simulink model "stm32f4_ds3231_read_temperature_demo"  (Simulink 7.3)
settings: Solver=FixedStepDiscrete  SolverMode=SingleTasking  StartTime=0.0  StopTime=10.0  RelTol=1e-3
PreLoadFcn:
  | waijung.modelPreload; % Required for working with Waijung Blockset. Do not remove.
undefined symbols (not defined in the file): HSEOSC, Link, LQFP176, ST, STM32F417IG
libraries: simulink x5, stm32f4_device_config_lib x1
CloseFcn:
  | waijung.modelClose; % Required for working with Waijung Blockset. Do not remove.
settings Model: Creator=Krisada  LastModifiedBy=Krisada
settings OptimizationCC: OptimizeModelRefInitCode=on  LifeSpan=1
settings HardwareCC: ProdEndianess=LittleEndian  ProdHWDeviceType=ARM Compatible->Cortex - M4  TargetEndianess=LittleEndian  TargetHWDeviceType=ARM Compatible->Cortex - M4
settings RTWCC: SystemTargetFile=stm32f4.tlc  GenerateMakefile=off  TemplateMakefile=ert_default_tmf  Description=STM32F4 Target  ProcessScript=stm32f4_make_rtw_hook
settings CodeAppCC: IgnoreCustomStorageClasses=off
settings STFCustomTargetCC: ModelReferenceCompliant=off  CombineOutputUpdateFcns=on  ERTCustomFileBanners=on  SupportContinuousTime=off  SupportNonInlinedSFcns=off  SystemTargetFile=stm32f4.tlc
settings ERTTargetCC: MultiwordLength=2048  ModelReferenceCompliant=off  ParMdlRefBuildCompliant=off  CompOptLevelCompliant=off  ERTFirstTimeCompliant=off  ModelStepFunctionPrototypeControlCompliant=off  CPPClassGenCompliant=off  ExtModeMexFile=noextcomm  InlinedParameterPlacement=NonHierarchical  ERTSrcFileBannerTemplate=stm32f4_code_template.cgt  ERTHdrFileBannerTemplate=stm32f4_code_template.cgt  ERTDataSrcFileTemplate=stm32f4_code_template.cgt  ERTDataHdrFileTemplate=stm32f4_code_template.cgt  ERTCustomFileTemplate=stm32f4_file_process.tlc

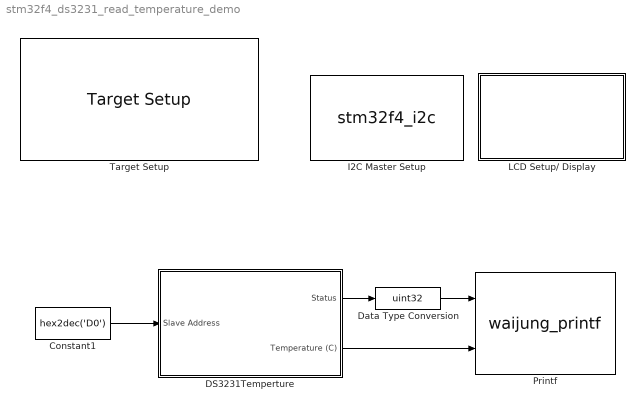
== system stm32f4_ds3231_read_temperature_demo ==
  Constant1 : Constant  Value=hex2dec('D0')  OutDataTypeMode=uint8  OutDataType=fixdt(1, 16)  OutScaling=2^0  OutDataTypeStr=uint8  SampleTime=0.5
  DS3231Temperture : Subsystem  mask{blockfunction=temp, module=1}
      mask prompts: blockfunction "Function"; module "I2C module"
      mask help:
      | The block implement temperature reading from DS3231 (Extremely Accurate RTC).
      | Its override the CONV bit, to force the temperature update, so the recommend sample time for this block is more than 0.5 seconds.
      | To get reading value from DS3231 device, this block generate 3 transaction of I2C as below:
      | 1. Read 2 bytes data from register 0x11 and 0x12 (Sequential read).
      | 2. Read 1 byte data from register 0x0F (Status) for poll BSY bit.
      | 3. Write 1 byte data to register 0x0E to force temperature conversion, CONV bit.
      mask init:
      | amg_high_precision_rtc_callback('init');
      mask StyleString: popup(temp|time|date),popup(1|2|3)
      mask CallbackString: |amg_high_precision_rtc_callback('module');
      mask Display: text(0.5, 0.5, 'Port: I2C1','ver','middle','hor','center');port_label('input', 1,'SlvAddr');port_label('output', 1,'Status');port_label('output', 2,'Temp (C)');
  Data Type Conversion : DataTypeConversion  OutDataTypeMode=uint32  OutDataType=fixdt(1, 16)  OutScaling=2^0  OutDataTypeStr=uint32
  I2C Master Setup : S-Function  FunctionName=stm32f4_i2c  Parameters=configuration,module,transfer,clkspeed,timeout,sdapin,sclpin,writecount,readcount,inputtypearray,outputtypearray,confstr,sampletime,sampletimestr,blockid  EnableBusSupport=off  mask(stm32f4_i2c){configuration=Setup, module=1, lastmodule=1, transfer=Blocking, dutycycle=TLow/THigh = 2, clkspeed=400, timeout=25, writecount=0, readcount=0, sdapin=B7, sclpin=B6, waitwritetime=0, inputtypearray=[0], outputtypearray=[0], confstr=["B","7","B","6","1","1","6","0","I2C_DutyCycle_2","0","off"], sampletime=-1, sampletimestr=0.01, blockid=I2CMasterSetup}
      mask prompts: module "I2C Module"; lastmodule "Last module"; transfer "Transfer mode"; dutycycle "Duty cycle in fast mode"; clkspeed "Clock speed (kHz)"; timeout "Timeout (ms)"; writecount "Bytes write count"; readcount "Bytes read count"; sdapin "SDA pin"; sclpin "SCL pin"; waitwritetime "Wait write time (ms), default is 0"; inputtypearray "Input type array"; outputtypearray "Output type array"; confstr "Configuration string"; sampletime "Sample time (sec)"; sampletimestr "Compiled sample time (sec) in string"
      mask init:
      | stm32f4_i2c_callback('init');
      mask Help: web(fullfile(waijungdocroot,'stm32f4_i2c_setup.htm'), '-browser')
      mask StyleString: popup(Setup|Transaction),popup(1|2|3),edit,popup(Blocking|Non-blocking),popup(TLow/THigh = 16/9|TLow/THigh = 2),edit,edit,edit,edit,popup(Not used|B7|B9),popup(Not used|B6|B8),edit,edit,edit,edit,edit,edit,edit
      mask CallbackString: stm32f4_i2c_callback('configuration');|stm32f4_i2c_callback('module');|||stm32f4_i2c_callback('dutycycle');|||stm32f4_i2c_callback('writecount');|stm32f4_i2c_callback('readcount');|stm32f4_i2c_callback('sdapin');|stm32f4_i2c_callback('sclpin');||||stm32f4_i2c_callback('confstr');|stm32f4_i2c_callback('sampletime');|stm32f4_i2c_callback('sampletimestr');|stm32f4_i2c_callback('blockid');
      mask Display: text(0.5, 0.5, 'Module: I2C1\nClock: 400kHz\nSDA/SCL Pin: B7/B6','ver','middle','hor','center');
  LCD Setup/ Display : Subsystem
  Printf : S-Function  FunctionName=waijung_printf  Parameters=storagename,printfformat,formatcode,varname,sampletime,sampletimestr,blockid  EnableBusSupport=off  mask(waijung_printf){storagename=S, printfformat=Status:%u, %1.2fC, formatcode=uf, varname=LCDSetupDisplayVolatileDataStorage_S, sampletime=-1, sampletimestr=0.5, blockid=Printf}
      mask prompts: storagename "Storage Name"; printfformat "Printf format"; formatcode "Printf format code"; varname "Variable name"; sampletime "Sample time (sec)"; sampletimestr "Compiled sample time (sec) in string"
      mask help: This block implements printf command.
      mask init:
      | waijung_printf_callback('init');
      mask Help: web(fullfile(waijungdocroot,'waijung_printf.htm'))
      mask StyleString: popup(S),edit,edit,edit,edit,edit,edit
      mask CallbackString: waijung_printf_callback('storagename');|waijung_printf_callback('printfformat');|waijung_printf_callback('formatcode');|waijung_printf_callback('varname');|waijung_printf_callback('sampletime');|waijung_printf_callback('sampletimestr');|waijung_printf_callback('blockid');
      mask Display: text(0.95, 0.5, 'Buffer: S\nTs (sec): 0.5','ver','middle','hor','right');port_label('input',1,'D1(%u)');port_label('input',2,'D2(%f)');
  Target Setup : stm32f4_device_config_lib/Target Setup  Priority=100  compiler=GNU ARM  previous_compiler=GNU ARM  mcu=STM32F417IG (LQFP176)  mcustr=STM32F417IG  clockconfig=HSEOSC-8MHz  system_stm32f4xx_c_path=F:\trunk\targets\stm32f4_target\stm32f4\utils\system_stm32f4xx_default\STM32F40_41xxx\hseosc8mhz  showmemoryconfiguration=off  stacksize=0x400  heapsize=0x200  enableautocompiledownload=on  fullchiperase=off  programmerinterface=ST-Link  editctrlstr=on  compilercontrolstr=$(patsubst %, -I%, .) -mcpu=cortex-m4 -mthumb -mthumb-interwork -mfloat-abi=hard -mfpu=fpv4-sp-d16 -ffast-math -Wall -Wextra -Ofast  assemblercontrolstr=$(patsubst %, -I%, .) -mcpu=cortex-m4 -mthumb -mthumb-interwork -mfloat-abi=hard -mfpu=fpv4-sp-d16 -ffast-math -Wall -Wextra -Ofast -Wa,-amhls=$(<:.s=.lst) -D__STACK_SIZE=$(STACK_SIZE) -D__HEAP_SIZE=$(HEAP_SIZE)  linkercontrolstr=-T$(LD_SCRIPT) -g -Wl,-Map=$(MAP),--cref,--no-warn-mismatch -mcpu=cortex-m4 -mthumb -mthumb-interwork -mfloat-abi=hard -mfpu=fpv4-sp-d16 -specs=nosys.specs  runafterdownload=on  execprofile=None  profileruart=1  profilerbaud=115200  profilertxpin=D8  profilerinitstr=0.01,168000000,1680000,115200,0  manualsetsampletime=off  sampletime=0.01  blockid=TargetSetup  systickreloadvalue=1680000  hseval=8000000  lastprofileruart=1  hclk=168000000  flashorigin=0x8000000  flashlength=1024k  ramorigin=0x20000000  ramlength=128k  useextram=off
  wires:
  Data Type Conversion/1 -> Printf/1
  DS3231Temperture/2(Temperature (C)) -> Printf/2
  DS3231Temperture/1(Status) -> Data Type Conversion/1
  Constant1/1 -> DS3231Temperture/1(Slave Address)

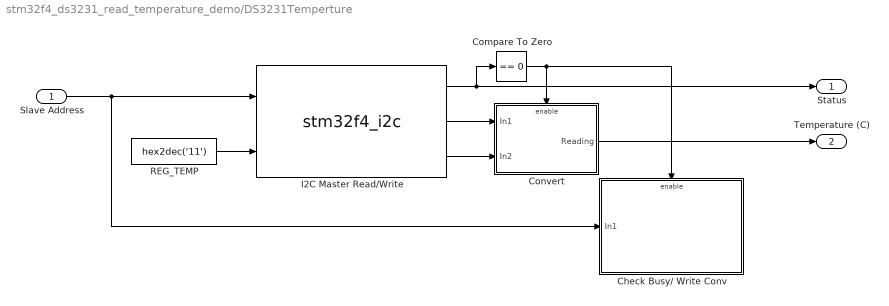
== system stm32f4_ds3231_read_temperature_demo/DS3231Temperture ==
  Slave Address : Inport  OutDataType=fixdt(1, 16)  OutScaling=2^0
  Check Busy/ Write Conv : Subsystem
  Compare To Zero : simulink/Logic and Bit Operations/Compare To Zero  SystemSampleTime=-1  relop===  LogicOutDataTypeMode=uint8  ZeroCross=off
  Convert : Subsystem  TreatAsAtomicUnit=on
  I2C Master Read/Write : S-Function  FunctionName=stm32f4_i2c  Parameters=configuration,module,transfer,clkspeed,timeout,sdapin,sclpin,writecount,readcount,inputtypearray,outputtypearray,confstr,sampletime,sampletimestr,blockid  EnableBusSupport=off  mask(stm32f4_i2c){configuration=Transaction, module=1, lastmodule=3, transfer=Blocking, dutycycle=TLow/THigh = 2, clkspeed=400, timeout=25, writecount=1, readcount=2, sdapin=C9, sclpin=A8, waitwritetime=0, inputtypearray=[2 3 3], outputtypearray=[3 3 3 3], confstr=["C","9","A","8","1","1","6","0","I2C_DutyCycle_2","0","off"], sampletime=-1, sampletimestr=0.5, blockid=DS3231TempertureI2CMasterReadWrite}
      mask prompts: module "I2C Module"; lastmodule "Last module"; transfer "Transfer mode"; dutycycle "Duty cycle in fast mode"; clkspeed "Clock speed (kHz)"; timeout "Timeout (ms)"; writecount "Bytes write count"; readcount "Bytes read count"; sdapin "SDA pin"; sclpin "SCL pin"; waitwritetime "Wait write time (ms), default is 0"; inputtypearray "Input type array"; outputtypearray "Output type array"; confstr "Configuration string"; sampletime "Sample time (sec)"; sampletimestr "Compiled sample time (sec) in string"
      mask init:
      | stm32f4_i2c_callback('init');
      mask Help: web(fullfile(waijungdocroot,'stm32f4_i2c_readwrite.htm'), '-browser')
      mask StyleString: popup(Setup|Transaction),popup(1|2|3),edit,popup(Blocking|Non-blocking),popup(TLow/THigh = 16/9|TLow/THigh = 2),edit,edit,edit,edit,popup(-|C9),popup(-|A8),edit,edit,edit,edit,edit,edit,edit
      mask CallbackString: stm32f4_i2c_callback('configuration');|stm32f4_i2c_callback('module');|||stm32f4_i2c_callback('dutycycle');|||stm32f4_i2c_callback('writecount');|stm32f4_i2c_callback('readcount');|stm32f4_i2c_callback('sdapin');|stm32f4_i2c_callback('sclpin');||||stm32f4_i2c_callback('confstr');|stm32f4_i2c_callback('sampletime');|stm32f4_i2c_callback('sampletimestr');|stm32f4_i2c_callback('blockid');
      mask Display: text(0.5, 0.5, 'Module: I2C1\nTransfer: Blocking\nWrite: 1 bytes\nRead: 2 bytes\nTs (sec): 0.5','ver','middle','hor','center');port_label('input', 1,'SlvAddr');port_label('input', 2,'Wr0 (uint8)');port_label('output', 1,'Status');port_label('output', 2,'Rd0 (uint8)');port_label('output', 3,'Rd1 (uint8)');
  REG_TEMP : Constant  Value=hex2dec('11')  OutDataTypeMode=uint8  OutDataType=fixdt(1, 16)  OutScaling=2^0  OutDataTypeStr=uint8
  Status : Outport
  Temperature (C) : Outport  Port=2
  wires:
  Convert/1(Reading) -> Temperature (C)/1
  I2C Master Read/Write/3 -> Convert/2(In2)
  I2C Master Read/Write/2 -> Convert/1(In1)
  Compare To Zero/1 -> Check Busy/ Write Conv/Enable, Convert/Enable
  I2C Master Read/Write/1 -> Compare To Zero/1, Status/1
  REG_TEMP/1 -> I2C Master Read/Write/2
  Slave Address/1 -> Check Busy/ Write Conv/1(In1), I2C Master Read/Write/1

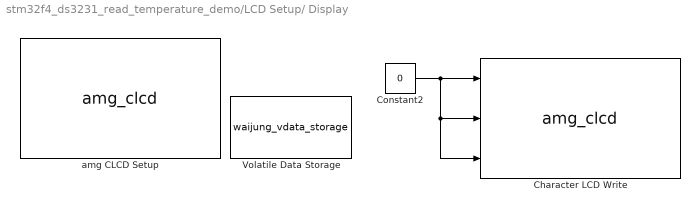
== system stm32f4_ds3231_read_temperature_demo/LCD Setup/ Display ==
  Character LCD Write : S-Function  FunctionName=amg_clcd  Parameters=module,configuration,inputtypearray,outputtypearray,confstr,sampletime,sampletimestr,blockid  EnableBusSupport=off  mask(amg_clcd){configuration=Transaction, module=1, model=amg CLCD Std, interface=4-bits, linecount=4, columncount=20, gpiotype=Push-pull, controlport=E, control_rs=15, control_rw=13, control_en=11, dataport=A, data0=7, data1=5, data2=3, data3=1, usestringbuffer=on, stringbuffer=S, varname=LCDSetupDisplayVolatileDataStorage_S, inputtypearray=[3 -1 -1 -1], outputtypearray=[0], confstr=["4","4","20","PP","E","15","11","13","","A","","","","","7","5","3","1","1","LCDSetupDisplayVolatileDataStorage_S","1","0","0","0","1","0","0","0","0","stm32f4"], sampletime=-1, sampletimestr=0.01, blockid=LCDSetupDisplayCharacterLCDWrite}
      mask prompts: model "LCD model:"; linecount "Number of lines:"; columncount "Number of columns:"; gpiotype "GPIO Output type:"; controlport "GPIO control port:"; control_rs "GPIO control pin, RS:"; control_rw "GPIO control pin, RW:"; control_en "GPIO control pin, EN:"; dataport "GPIO data D[7:4] port"; data0 "GPIO data pin, D4:"; data1 "GPIO data pin, D5:"; data2 "GPIO data pin, D6:"; data3 "GPIO data pin, D7:"; usestringbuffer "Use string buffer"; stringbuffer "String buffer"; varname "Variable name"; inputtypearray "Input type array"; outputtypearray "Output type array"; confstr "Configuration string"; sampletime "Sample time (sec)"; sampletimestr "Compiled sample time (sec) in string"
      mask help:
      | Note for cmd:
      | 1 - Clear LCD Line before write.
      | 0 or otherwise - Write into LCD Line with existing data.
      mask init:
      | amg_clcd_callback('init');
      mask Help: web(fullfile(waijungdocroot,'amg_clcd_write.htm'), '-browser')
      mask StyleString: popup(Setup|Transaction),popup(1|2|3|4),popup(amg CLCD Std),popup(4-bits),edit,edit,popup(Push-pull|Open-drain),popup(A|B|C|D|E|F|G|H|I),popup(0|1|2|3|4|5|6|7|8|9|10|11|12|13|14|15),popup(0|1|2|3|4|5|6|7|8|9|10|11|12|13|14|15),popup(0|1|2|3|4|5|6|7|8|9|10|11|12|13|14|15),popup(A|B|C|D|E|F|G|H|I),popup(0|1|2|3|4|5|6|7|8|9|10|11|12|13|14|15),popup(0|1|2|3|4|5|6|7|8|9|10|11|12|13|14|15),popup(0|1|2|3|4|5|6|7|8|9|10|11|12|13|14|15),popup(0|1|2|3|4|5|6|7|8|9|10|11|12|13|14|15),checkbox,popup(S),edit,edit,edit,edit,edit,edit,edit
      mask CallbackString: amg_clcd_callback('configuration');||||||||||||||||amg_clcd_callback('usestringbuffer');||amg_clcd_callback('varname');|||amg_clcd_callback('confstr');|amg_clcd_callback('sampletime');|amg_clcd_callback('sampletimestr');|amg_clcd_callback('blockid');
      mask Display: text(0.5, 0.5, 'Module: CLCD1 (Write)\nBuffer: S\nTs (sec): 0.01','ver','middle','hor','center');port_label('input', 1,'cmd');port_label('input', 2,'xpos');port_label('input', 3,'ypos');
  Constant2 : Constant  Value=0  OutDataTypeMode=uint8  OutDataType=fixdt(1, 16)  OutScaling=2^0  OutDataTypeStr=uint8
  Volatile Data Storage : S-Function  FunctionName=waijung_vdata_storage  Parameters=storagetype,storagename,initval,varname,buffersize,initvalstring,sampletime,sampletimestr,blockid,storagetypestr  EnableBusSupport=off  mask(waijung_vdata_storage){storagetype=string, storagename=S, initval=0, varname=LCDSetupDisplayVolatileDataStorage_S, buffersize=64, initvalstring='', webintegration=Disable, weboutputformat='%s', webcgicallback=(void*)0, laststoragetype=string, sampletime=-1, sampletimestr=0.01, blockid=LCDSetupDisplayVolatileDataStorage, storagetypestr=char}
      mask prompts: storagetype "Storage Type"; storagename "Storage Name (must be a valid variable name)"; initval "Initial value (Apply at Power on Reset only)"; varname "Variable name"; buffersize "Size (bytes)"; initvalstring "Initial value (Apply at Power on Reset only)"; webintegration "Web CGI varget/varset integration"; weboutputformat "Web CGI varget output format"; webcgicallback "Web CGI varset callback"; laststoragetype "Last selected Storage Type"; sampletime "Sample time (sec)"; sampletimestr "Compiled sample time (sec) in string"; storagetypestr "Type string"
      mask help:
      | This block implements a volatile Data Storage.
      |
      | Web CGI varset/varget integratiopn:
      | Enable - In webserver application, allow remote access via http.
      | Disable - Variable is use in local only.
      mask init:
      | waijung_vdata_storage_callback('init');
      mask Help: web(fullfile(waijungdocroot,'Volatile_Data_Storage.htm'))
      mask StyleString: popup(double|single|uint32|int32|uint16|int16|uint8|int8|string),edit,edit,edit,edit,edit,popup(Disable|ReadOnly|Write/ Read|ReadOnly with KeyValuePair|Write/ Read with KeyValuePair),edit,edit,popup(double|single|uint32|int32|uint16|int16|uint8|int8|string),edit,edit,edit,edit
      mask CallbackString: waijung_vdata_storage_callback('storagetype');|waijung_vdata_storage_callback('storagename');|waijung_vdata_storage_callback('initval');|waijung_vdata_storage_callback('varname');||waijung_vdata_storage_callback('initvalstring');|waijung_vdata_storage_callback('webintegration');|waijung_vdata_storage_callback('weboutputformat');|||waijung_vdata_storage_callback('sampletime');|waijung_vdata_storage_callback('sampletimestr');|waijung_vdata_storage_callback('blockid');|
      mask Display: text(0.5, 0.5, 'Name: S\nType: string','ver','middle','hor','center')
  amg CLCD Setup : S-Function  FunctionName=amg_clcd  Parameters=module,configuration,inputtypearray,outputtypearray,confstr,sampletime,sampletimestr,blockid  EnableBusSupport=off  mask(amg_clcd){configuration=Setup, module=1, model=amg CLCD Std, interface=4-bits, linecount=4, columncount=16, gpiotype=Push-pull, controlport=E, control_rs=7, control_rw=8, control_en=9, dataport=E, data0=12, data1=13, data2=14, data3=15, usestringbuffer=off, stringbuffer=Line2, varname=clcd_demo_4linesLCDSetupVolatileDataStorage3_Line2, inputtypearray=[0], outputtypearray=[0], confstr=["4","4","16","PP","E","7","9","8","","E","","","","","12","13","14","15","0","","0","0","0","0","1","0","0","0","0","stm32f4"], sampletime=-1, sampletimestr=0.01, blockid=LCDSetupDisplayamgCLCDSetup}
      mask prompts: model "LCD model:"; linecount "Number of lines:"; columncount "Number of columns:"; gpiotype "GPIO Pull-Up/Down:"; controlport "GPIO control port:"; control_rs "GPIO control pin, RS:"; control_rw "GPIO control pin, RW:"; control_en "GPIO control pin, EN:"; dataport "GPIO data D[7:4] port"; data0 "GPIO data pin, D4:"; data1 "GPIO data pin, D5:"; data2 "GPIO data pin, D6:"; data3 "GPIO data pin, D7:"; usestringbuffer "Use string buffer"; stringbuffer "String buffer"; varname "Variable name"; inputtypearray "Input type array"; outputtypearray "Output type array"; confstr "Configuration string"; sampletime "Sample time (sec)"; sampletimestr "Compiled sample time (sec) in string"
      mask init:
      | amg_clcd_callback('init');
      mask Help: web(fullfile(waijungdocroot,'amg_clcd_setup.htm'), '-browser')
      mask StyleString: popup(Setup|Transaction),popup(1|2|3|4),popup(amg CLCD Std),popup(4-bits),edit,edit,popup(Push-pull|Open-drain),popup(A|B|C|D|E|F|G|H|I),popup(0|1|2|3|4|5|6|7|8|9|10|11|12|13|14|15),popup(0|1|2|3|4|5|6|7|8|9|10|11|12|13|14|15),popup(0|1|2|3|4|5|6|7|8|9|10|11|12|13|14|15),popup(A|B|C|D|E|F|G|H|I),popup(0|1|2|3|4|5|6|7|8|9|10|11|12|13|14|15),popup(0|1|2|3|4|5|6|7|8|9|10|11|12|13|14|15),popup(0|1|2|3|4|5|6|7|8|9|10|11|12|13|14|15),popup(0|1|2|3|4|5|6|7|8|9|10|11|12|13|14|15),checkbox,popup(Line3|Line1|Line2|Line4),edit,edit,edit,edit,edit,edit,edit
      mask CallbackString: amg_clcd_callback('configuration');||||||||||||||||amg_clcd_callback('usestringbuffer');||amg_clcd_callback('varname');|||amg_clcd_callback('confstr');|amg_clcd_callback('sampletime');|amg_clcd_callback('sampletimestr');|amg_clcd_callback('blockid');
      mask Display: text(0.5, 0.5, 'Module: CLCD1 (Setup)\nInterface: 4-bits\nCntrl: E7/E8/E9\nD[7:4]: E12/E13/E14/E15\nTs (sec): 0.01','ver','middle','hor','center');
  wires:
  Constant2/1 -> Character LCD Write/1, Character LCD Write/2, Character LCD Write/3

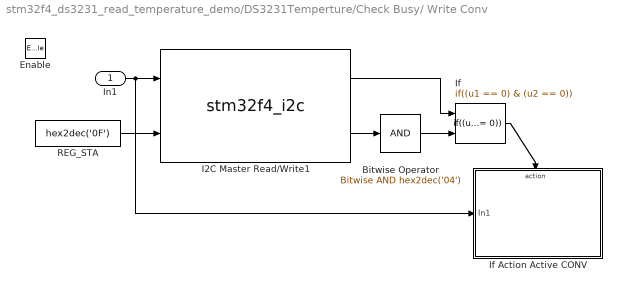
== system stm32f4_ds3231_read_temperature_demo/DS3231Temperture/Check Busy/ Write Conv ==
  In1 : Inport
  Enable : EnablePort
  Bitwise Operator : simulink/Logic and Bit Operations/Bitwise Operator  logicop=AND  UseBitMask=on  BitMask=hex2dec('04')  BitMaskRealWorld=Stored Integer
  I2C Master Read/Write1 : S-Function  FunctionName=stm32f4_i2c  Parameters=configuration,module,transfer,clkspeed,timeout,sdapin,sclpin,writecount,readcount,inputtypearray,outputtypearray,confstr,sampletime,sampletimestr,blockid  EnableBusSupport=off  mask(stm32f4_i2c){configuration=Transaction, module=1, lastmodule=3, transfer=Blocking, dutycycle=TLow/THigh = 2, clkspeed=400, timeout=25, writecount=1, readcount=1, sdapin=C9, sclpin=A8, waitwritetime=0, inputtypearray=[2 3 3], outputtypearray=[2 3 3], confstr=["C","9","A","8","1","1","6","0","I2C_DutyCycle_2","0","off"], sampletime=-1, sampletimestr=0.5, blockid=DS3231TempertureCheckBusyWriteConvI2CMasterReadWrite1}
      mask prompts: module "I2C Module"; lastmodule "Last module"; transfer "Transfer mode"; dutycycle "Duty cycle in fast mode"; clkspeed "Clock speed (kHz)"; timeout "Timeout (ms)"; writecount "Bytes write count"; readcount "Bytes read count"; sdapin "SDA pin"; sclpin "SCL pin"; waitwritetime "Wait write time (ms), default is 0"; inputtypearray "Input type array"; outputtypearray "Output type array"; confstr "Configuration string"; sampletime "Sample time (sec)"; sampletimestr "Compiled sample time (sec) in string"
      mask init:
      | stm32f4_i2c_callback('init');
      mask Help: web(fullfile(waijungdocroot,'stm32f4_i2c_readwrite.htm'), '-browser')
      mask StyleString: popup(Setup|Transaction),popup(1|2|3),edit,popup(Blocking|Non-blocking),popup(TLow/THigh = 16/9|TLow/THigh = 2),edit,edit,edit,edit,popup(-|C9),popup(-|A8),edit,edit,edit,edit,edit,edit,edit
      mask CallbackString: stm32f4_i2c_callback('configuration');|stm32f4_i2c_callback('module');|||stm32f4_i2c_callback('dutycycle');|||stm32f4_i2c_callback('writecount');|stm32f4_i2c_callback('readcount');|stm32f4_i2c_callback('sdapin');|stm32f4_i2c_callback('sclpin');||||stm32f4_i2c_callback('confstr');|stm32f4_i2c_callback('sampletime');|stm32f4_i2c_callback('sampletimestr');|stm32f4_i2c_callback('blockid');
      mask Display: text(0.5, 0.5, 'Module: I2C1\nTransfer: Blocking\nWrite: 1 bytes\nRead: 1 bytes\nTs (sec): 0.5','ver','middle','hor','center');port_label('input', 1,'SlvAddr');port_label('input', 2,'Wr0 (uint8)');port_label('output', 1,'Status');port_label('output', 2,'Rd0 (uint8)');
  If : If  NumInputs=2  IfExpression=(u1 == 0) & (u2 == 0)  ShowElse=off
  If Action Active CONV : Subsystem  TreatAsAtomicUnit=on
  REG_STA : Constant  Value=hex2dec('0F')  OutDataTypeMode=uint8  OutDataType=fixdt(1, 16)  OutScaling=2^0  OutDataTypeStr=uint8
  wires:
  If/1 -> If Action Active CONV/Action
  Bitwise Operator/1 -> If/2
  I2C Master Read/Write1/2 -> Bitwise Operator/1
  In1/1 -> If Action Active CONV/1(In1), I2C Master Read/Write1/1
  I2C Master Read/Write1/1 -> If/1
  REG_STA/1 -> I2C Master Read/Write1/2

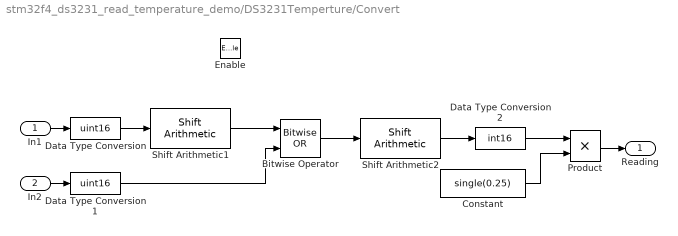
== system stm32f4_ds3231_read_temperature_demo/DS3231Temperture/Convert ==
  In1 : Inport  OutDataType=fixdt(1, 16)  OutScaling=2^0
  In2 : Inport  Port=2  OutDataType=fixdt(1, 16)  OutScaling=2^0
  Enable : EnablePort
  Bitwise Operator : simulink/Logic and Bit Operations/Bitwise Operator  logicop=OR  UseBitMask=off  NumInputPorts=2  BitMask=bin2dec('11011001')  BitMaskRealWorld=Stored Integer
  Constant : Constant  Value=single(0.25)  OutDataType=fixdt(1, 16)  OutScaling=2^0
  Data Type Conversion : DataTypeConversion  OutDataTypeMode=uint16  OutDataType=fixdt(1, 16)  OutScaling=2^0  OutDataTypeStr=uint16
  Data Type Conversion1 : DataTypeConversion  OutDataTypeMode=uint16  OutDataType=fixdt(1, 16)  OutScaling=2^0  OutDataTypeStr=uint16
  Data Type Conversion2 : DataTypeConversion  OutDataTypeMode=int16  OutDataType=fixdt(1, 16)  OutScaling=2^0  OutDataTypeStr=int16
  Product : Product  OutDataTypeMode=single  OutDataType=fixdt(1, 16)  OutScaling=2^0  OutDataTypeStr=single  RndMeth=Zero
  Shift Arithmetic1 : simulink/Logic and Bit Operations/Shift Arithmetic  SystemSampleTime=-1  nBitShiftRight=-8  nBinPtShiftRight=0
  Shift Arithmetic2 : simulink/Logic and Bit Operations/Shift Arithmetic  SystemSampleTime=-1  nBitShiftRight=6  nBinPtShiftRight=0
  Reading : Outport  OutDataType=fixdt(1, 16)  OutScaling=2^0
  wires:
  Shift Arithmetic2/1 -> Data Type Conversion2/1
  Product/1 -> Reading/1
  Constant/1 -> Product/2
  Data Type Conversion2/1 -> Product/1
  Bitwise Operator/1 -> Shift Arithmetic2/1
  Data Type Conversion1/1 -> Bitwise Operator/2
  Shift Arithmetic1/1 -> Bitwise Operator/1
  Data Type Conversion/1 -> Shift Arithmetic1/1
  In2/1 -> Data Type Conversion1/1
  In1/1 -> Data Type Conversion/1

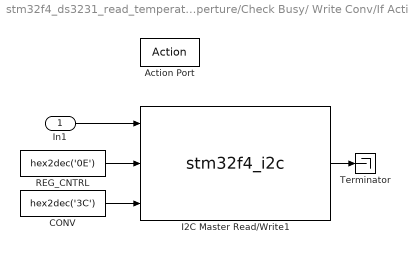
== system stm32f4_ds3231_read_temperature_demo/DS3231Temperture/Check Busy/ Write Conv/If Action Active CONV ==
  In1 : Inport  OutDataType=fixdt(1, 16)  OutScaling=2^0
  Action Port : ActionPort  ActionType=then
  CONV : Constant  Value=hex2dec('3C')  OutDataTypeMode=uint8  OutDataType=fixdt(1, 16)  OutScaling=2^0  OutDataTypeStr=uint8
  I2C Master Read/Write1 : S-Function  FunctionName=stm32f4_i2c  Parameters=configuration,module,transfer,clkspeed,timeout,sdapin,sclpin,writecount,readcount,inputtypearray,outputtypearray,confstr,sampletime,sampletimestr,blockid  EnableBusSupport=off  mask(stm32f4_i2c){configuration=Transaction, module=1, lastmodule=3, transfer=Blocking, dutycycle=TLow/THigh = 2, clkspeed=400, timeout=25, writecount=2, readcount=0, sdapin=C9, sclpin=A8, waitwritetime=0, inputtypearray=[3 3 3 3], outputtypearray=[1 3], confstr=["C","9","A","8","1","1","6","0","I2C_DutyCycle_2","0","off"], sampletime=-1, sampletimestr=0.5, blockid=DS3231TempertureCheckBusyWriteConvIfActionActiveCONVI2CMasterReadWrite1}
      mask prompts: module "I2C Module"; lastmodule "Last module"; transfer "Transfer mode"; dutycycle "Duty cycle in fast mode"; clkspeed "Clock speed (kHz)"; timeout "Timeout (ms)"; writecount "Bytes write count"; readcount "Bytes read count"; sdapin "SDA pin"; sclpin "SCL pin"; waitwritetime "Wait write time (ms), default is 0"; inputtypearray "Input type array"; outputtypearray "Output type array"; confstr "Configuration string"; sampletime "Sample time (sec)"; sampletimestr "Compiled sample time (sec) in string"
      mask init:
      | stm32f4_i2c_callback('init');
      mask Help: web(fullfile(waijungdocroot,'stm32f4_i2c_readwrite.htm'), '-browser')
      mask StyleString: popup(Setup|Transaction),popup(1|2|3),edit,popup(Blocking|Non-blocking),popup(TLow/THigh = 16/9|TLow/THigh = 2),edit,edit,edit,edit,popup(-|C9),popup(-|A8),edit,edit,edit,edit,edit,edit,edit
      mask CallbackString: stm32f4_i2c_callback('configuration');|stm32f4_i2c_callback('module');|||stm32f4_i2c_callback('dutycycle');|||stm32f4_i2c_callback('writecount');|stm32f4_i2c_callback('readcount');|stm32f4_i2c_callback('sdapin');|stm32f4_i2c_callback('sclpin');||||stm32f4_i2c_callback('confstr');|stm32f4_i2c_callback('sampletime');|stm32f4_i2c_callback('sampletimestr');|stm32f4_i2c_callback('blockid');
      mask Display: text(0.5, 0.5, 'Module: I2C1\nTransfer: Blocking\nWrite: 2 bytes\nRead: 0 bytes\nTs (sec): 0.5','ver','middle','hor','center');port_label('input', 1,'SlvAddr');port_label('input', 2,'Wr0 (uint8)');port_label('input', 3,'Wr1 (uint8)');port_label('output', 1,'Status');
  REG_CNTRL : Constant  Value=hex2dec('0E')  OutDataTypeMode=uint8  OutDataType=fixdt(1, 16)  OutScaling=2^0  OutDataTypeStr=uint8
  Terminator : Terminator
  wires:
  I2C Master Read/Write1/1 -> Terminator/1
  REG_CNTRL/1 -> I2C Master Read/Write1/2
  CONV/1 -> I2C Master Read/Write1/3
  In1/1 -> I2C Master Read/Write1/1
